simulink model "LKAS"  (R2018b)
settings: Solver=FixedStepDiscrete  StartTime=0.0  StopTime=10.0  FixedStep=0.01  RelTol=1e-3
InitFcn:
  | tmpVer = ver('MATLAB');
  | tmpVer = str2num(tmpVer.Version);
  | % -------------------------------------------------------------------
  | %  MATLAB file generated by Simulink.saveVars on 21-Nov-2019 10:06:14
  | %  MATLAB version: 7.13.0.564 (R2011b)
  | % -------------------------------------------------------------------
  | 
  | 
  | SInt16 = Simulink.AliasType;
  | SInt16.Description = 'Num';
  | if (tmpVer > 7.11)
  | 	SInt16.DataScope = 'Auto';
  | end
  | SInt16.HeaderFile = 'Rte_Type.h';
  | SInt16.BaseType = 'int16';
  | 
  | SInt32 = Simulink.AliasType;
  | SInt32.Description = 'Num';
  | if (tmpVer > 7.11)
  | 	SInt32.DataScope = 'Auto';
  | end
  | SInt32.HeaderFile = 'Rte_Type.h';
  | SInt32.BaseType = 'int32';
  | 
  | SInt8 = Simulink.AliasType;
  | SInt8.Description = 'Num';
  | if (tmpVer > 7.11)
  | 	SInt8.DataScope = 'Auto';
  | end
  | SInt8.HeaderFile = 'Rte_Type.h';
  | SInt8.BaseType = 'int8';
  | 
  | T_A_m2_1024_1_u32 = Simulink.NumericType;
  | T_A_m2_1024_1_u32.Description = 'm2 (square meters  (m2))';
  | if (tmpVer > 7.11)
  | 	T_A_m2_1024_1_u32.DataScope = 'Auto';
  | end
  | T_A_m2_1024_1_u32.HeaderFile = 'Rte_Type.h';
  | T_A_m2_1024_1_u32.DataTypeMode = 'Fixed-point: slope and bias scaling';
  | T_A_m2_1024_1_u32.SignednessBool = false;
  | T_A_m2_1024_1_u32.WordLength = 32;
  | T_A_m2_1024_1_u32.FixedExponent = -10;
  | T_A_m2_1024_1_u32.SlopeAdjustmentFactor = 1;
  | T_A_m2_1024_1_u32.Bias = 0;
  | T_A_m2_1024_1_u32.DataTypeOverride = 'Inherit';
  | T_A_m2_1024_1_u32.IsAlias = true;
  | 
  | T_A_m2_65536_1_u16 = Simulink.NumericType;
  | T_A_m2_65536_1_u16.Description = 'm2 (square meters  (m2))';
  | if (tmpVer > 7.11)
  | 	T_A_m2_65536_1_u16.DataScope = 'Auto';
  | end
  | T_A_m2_65536_1_u16.HeaderFile = 'Rte_Type.h';
  | T_A_m2_65536_1_u16.DataTypeMode = 'Fixed-point: slope and bias scaling';
  | T_A_m2_65536_1_u16.SignednessBool = false;
  | T_A_m2_65536_1_u16.WordLength = 16;
  | T_A_m2_65536_1_u16.FixedExponent = -16;
  | T_A_m2_65536_1_u16.SlopeAdjustmentFactor = 1;
  | T_A_m2_65536_1_u16.Bias = 0;
  | T_A_m2_65536_1_u16.DataTypeOverride = 'Inherit';
  | ... (+4598 lines)
StopFcn:
  | clear  T_A_m2_1024_1_u32 T_A_m2_65536_1_u16 T_A_m2_Float32 T_A_mm2_10_1_u16 T_A_mm2_4_1_s16 T_A_mm2_Float32 T_Cnt_Num_10_1_u32 T_Cnt_Num_1_1_s16 T_Cnt_Num_1_1_s32 T_Cnt_Num_1_1_s8 T_Cnt_Num_1_1_u16 T_Cnt_Num_1_1_u32 T_Cnt_Num_1_1_u8 T_E_J_1_1_s32 T_E_J_Float32 T_E_kJ_128_1_s32 T_E_kJ_Float32 T_E_kwh_10_1_u16 T_E_kwh_Float32 T_Epl_kwhpkm_100_1_u16 T_Epl_kwhpkm_Float32 T_F_N_1_1_s16 T_F_N_Float32 T_I_A_1000_1_u16 T_I_A_1048576_1_s32 T_I_A_2048_1_s16 T_I_A_32_1_s16 T_I_A_Float32 T_I_mA_1_1_s16 T_I_mA_32768_128_s16 T_I_mA_Float32 T_J_kgpm2_128_1_u16 T_J_kgpm2_Float32 T_K_NA_1000_1_s16 T_K_NA_100_1_s16 T_K_NA_100_1_u16 T_K_NA_1024_1_s16 T_K_NA_1024_1_u16 T_K_NA_128_1_s16 T_K_NA_128_1_u16 T_K_NA_128_1_u8 T_K_NA_16777216_1_u32 T_K_NA_16_1_s16 T_K_NA_16_1_u16 T_K_NA_16_1_u8 T_K_NA_1_16_u16 T_K_NA_1_1_s16 T_K_NA_1_1_u16 T_K_NA_1_1_u8 T_K_NA_32768_1_s16 T_K_NA_32768_1_u16 T_K_NA_32_1_s8 T_K_NA_4096_1_u16 T_K_NA_4194304_1_s32 T_K_NA_4194304_1_u16 T_K_NA_65536_1_s32 T_K_NA_65536_1_u16 T_K_NA_8192_1_s16 T_K_NA_8_1_s16 T_K_NA_Float32 T_M_Nm_16_1_s16 T_M_Nm_1_1_s16 T_M_Nm_32768_1_s16 T_M_Nm_32_1_s16 T_M_Nm_4_1_s16 T_M_Nm_512_1_s16 T_M_Nm_Float32 T_P_W_1_4_s16 T_P_W_1_8_s16 T_P_W_Float32 T_P_kW_128_1_s16 T_P_kW_1_8_s16 T_P_kW_8_1_s32 T_P_kW_Float32 T_Pct_pct_1024_1_s32 T_Pct_pct_1024_1_u32 T_Pct_pct_10_1_s16 T_Pct_pct_10_1_u32 T_Pct_pct_128_100_s8 T_Pct_pct_1_1_s16 T_Pct_pct_1_4_u8 T_Pct_pct_255_100_u16 T_Pct_pct_255_100_u8 T_Pct_pct_256_1_s16 T_Pct_pct_256_1_u16 T_Pct_pct_65535_100_u16 T_Pct_pct_Float32 T_R_ohm_1024_1_s16 T_R_ohm_32_1_s16 T_R_ohm_Float32 T_TK_K_16_1_s16 T_TK_K_Float32 T_T_degC_10_400_1_u16 T_T_degC_16_1_s16 T_T_degC_1_40_1_u8 T_T_degC_2_80_1_u8 T_T_degC_Float32 T_U_V_1000_1_u16 T_U_V_10_1_u8 T_U_V_200_1_u8 T_U_V_32_1_s16 T_U_V_4096_1_s16 T_U_V_512_1_s16 T_U_V_65535_8_u16 T_U_V_8192_1_u16 T_U_V_Float32 T_U_mV_1_1_s16 T_U_mV_256_20_u16 T_U_mV_Float32 T_V_l_256_1_s16 T_V_l_4096_1_s16 T_V_l_64_1_s16 T_V_l_65535_100_u16 T_V_l_Float32 T_V_ml_128_1_s16 T_V_ml_1_1_s16 T_V_ml_32768_1_s16 T_V_ml_Float32 T_V_ul_32_1_u16 T_V_ul_Float32 T_Vpl_clpkm_512_1_u16 T_Vpl_clpkm_Float32 T_a_kphps_16_1_s16 T_a_kphps_Float32 T_a_mps2_128_1_s16 T_a_mps2_Float32 T_c_MJpkg_256_1_s16 T_c_MJpkg_Float32 T_c_kJpgpK_1024_1_s16 T_c_kJpgpK_Float32 T_c_kJpkgpK_128_1_u16 T_c_kJpkgpK_Float32 T_chrg_Ah_1_1_s16 T_chrg_Ah_1_1_u16 T_chrg_Ah_1_1_u8 T_chrg_Ah_256_1_u16 T_chrg_Ah_4194304_1_s32 T_chrg_Ah_512_1_u16 T_chrg_Ah_8_1_u16 T_chrg_Ah_Float32 T_cmp_NA_100_1_s16 T_cmp_NA_128_1_s16 T_cmp_NA_16_1_s16 T_cmp_NA_32768_1_u16 T_cmp_NA_Float32 T_d2n_rpmps2_4_1_s16 T_d2n_rpmps2_Float32 T_dPct_pctps_16_1_s16 T_dPct_pctps_256_1_s16 T_dPct_pctps_Float32 T_dT_degCps_128_1_s16 T_dT_degCps_Float32 T_dV_lph_1_1_s16 T_dV_lph_Float32 T_dV_lpm_128_1_s16 T_dV_lpm_32_1_s16 T_dV_lpm_Float32 T_dV_lps_1024_1_u16 T_dV_lps_4_1_u16 T_dV_lps_Float32 T_dV_mlps_1024_1_s16 T_dV_mlps_Float32 T_d_BitField16 T_dm_gps_128_1_s16 T_dm_gps_128_1_u16 T_dm_gps_256_1_u16 T_dm_gps_Float32 T_dm_mgps_1_1_s16 T_dm_mgps_Float32 T_dn_rpmps_1_1_s16 T_dn_rpmps_2_1_s16 T_dn_rpmps_Float32 T_dp_Paps_1_1_s16 T_dp_Paps_Float32 T_dp_kPaps_1_1_s16 T_dp_kPaps_8_1_s16 T_dp_kPaps_Float32 T_dphi_degps_128_1_s16 T_dphi_degps_8_1_s16 T_dphi_degps_Float32 T_dr_ps_256_1_s16 T_dr_ps_Float32 T_drho_mgplps_1_2_s16 T_drho_mgplps_Float32 T_e_NA_1_1_u8 T_f_Hz_1_1_u16 T_f_Hz_1_1_u32 T_f_Hz_64_1_u16 T_f_Hz_8_1_s16 T_f_Hz_Float32 T_g_BitField32 T_l_km_16_1_s16 T_l_km_1_1_u16 T_l_km_1_1_u32 T_l_km_Float32 T_l_m_1024_1_s16 T_l_m_16_1_s16 T_l_m_1_1_u32 T_l_m_Float32 T_l_mm_16_1_s16 T_l_mm_1_1_u16 T_l_mm_4096_1_s16 T_l_mm_4_1_u8 T_l_mm_64_1_s16 T_l_mm_Float32 T_m_g_1_1_s16 T_m_g_2048_1_s16 T_m_g_32_1_u16 T_m_g_Float32 T_m_kg_1024_1_s16 T_m_kg_1_1_s16 T_m_kg_1_1_u32 T_m_kg_Float32 T_m_mg_128_1_s16 T_m_mg_32_1_s16 T_m_mg_Float32 T_n_rpm_1_1_s16 T_n_rpm_1_25_u8 T_n_rpm_256_50_u16 T_n_rpm_2_25_u8 T_n_rpm_4_1_u16 T_n_rpm_Float32 T_p_MPa_64_1_s16 T_p_MPa_Float32 T_p_Pa_1_1_s16 T_p_Pa_Float32 T_p_kPa_1_10_u16 T_p_kPa_1_1_s16 T_p_kPa_1_1_u8 T_p_kPa_256_1_u16 T_p_kPa_32_1_u16 T_p_kPa_64_1_s16 T_p_kPa_Float32 T_phi_deg_100_1_s16 T_phi_deg_1024_1_s16 T_phi_deg_128_1_s16 T_phi_deg_1_1_u8 T_phi_deg_256_1_s16 T_phi_deg_2_1_s8 T_phi_deg_32_1_s16 T_phi_deg_512_6_s32 T_phi_deg_Float32 T_phi_rad_2048_1_s16 T_phi_rad_Float32 T_r_NA_1024_1_s16 T_r_NA_1024_1_u16 T_r_NA_16384_1_s16 T_r_NA_16_1_s16 T_r_NA_256_1_s8 T_r_NA_256_1_u16 T_r_NA_32768_1_u16 T_r_NA_32_1_u16 T_r_NA_4096_1_s16 T_r_NA_65535_2_u16 T_r_NA_8192_1_u16 T_r_NA_Float32 T_rho_gpl_8192_1_s16 T_rho_gpl_Float32 T_rho_kgpm3_16_1_s16 T_rho_kgpm3_Float32 T_rho_mgpl_1_1_s16 T_rho_mgpl_64_1_s16 T_rho_mgpl_Float32 T_t_hour_1_1_s16 T_t_hour_Float32 T_t_m_1_1_u16 T_t_m_Float32 T_t_ms_1_1_s16 T_t_ms_1_1_u16 T_t_ms_1_1_u32 T_t_ms_4096_1_s16 T_t_ms_64_1_s16 T_t_ms_Float32 T_t_s_1000_1_s16 T_t_s_100_1_s16 T_t_s_10_1_s16 T_t_s_10_1_u16 T_t_s_1_1_s16 T_t_s_1_1_u16 T_t_s_1_1_u32 T_t_s_Float32 T_t_us_10_1_u32 T_t_us_1_1_s16 T_t_us_1_1_u32 T_t_us_1_4_u16 T_t_us_Float32 T_v_kph_1_1_u8 T_v_kph_64_1_s16 T_v_kph_64_1_u16 T_v_kph_Float32 T_v_mps_256_1_s16 T_v_mps_Float32 T_w_radps_32_1_s16 T_w_radps_Float32 T_y_BitField8 T_y_BitFieldDiagProgress T_y_BitFieldDiagStatus T_y_NA_1_1_u8 SInt16 SInt32 SInt8 T_BOOLEAN UInt16 UInt32 UInt8 s16 s32 s8 u16 u32 u8
model workspace (MAT data in the model file):
  MCOS : class17 (value not decoded)
  MCOS : class17 (value not decoded)
  MCOS : class17 (value not decoded)
  MCOS : class17 (value not decoded)
  MCOS : class17 (value not decoded)
  MCOS : class17 (value not decoded)
  MCOS : class17 (value not decoded)
  MCOS : class17 (value not decoded)
  MCOS : class17 (value not decoded)
  MCOS : class17 (value not decoded)
  MCOS : class17 (value not decoded)
  MCOS : class17 (value not decoded)
  MCOS : class17 (value not decoded)
  MCOS : class17 (value not decoded)
  MCOS : class17 (value not decoded)
  MCOS : class17 (value not decoded)
  MCOS : class17 (value not decoded)
  MCOS : class17 (value not decoded)
  MCOS : class17 (value not decoded)
  MCOS : class17 (value not decoded)
  MCOS : class17 (value not decoded)
  MCOS : class17 (value not decoded)
  MCOS : class17 (value not decoded)
  MCOS : class17 (value not decoded)
  MCOS : class17 (value not decoded)
  MCOS : class17 (value not decoded)
  MCOS : class17 (value not decoded)
  MCOS : class17 (value not decoded)
  MCOS : class17 (value not decoded)
  MCOS : class17 (value not decoded)
  MCOS : class17 (value not decoded)
  MCOS : class17 (value not decoded)
  MCOS : class17 (value not decoded)
  MCOS : class17 (value not decoded)
  MCOS : class17 (value not decoded)
  MCOS : class17 (value not decoded)
  MCOS : class17 (value not decoded)
  MCOS : class17 (value not decoded)
  MCOS : class17 (value not decoded)
  MCOS : class17 (value not decoded)
  MCOS : class17 (value not decoded)
  MCOS : class17 (value not decoded)
  MCOS : class17 (value not decoded)
  MCOS : class17 (value not decoded)
  MCOS : class17 (value not decoded)
  MCOS : class17 (value not decoded)
  MCOS : class17 (value not decoded)
  MCOS : class17 (value not decoded)
  MCOS : class17 (value not decoded)
  MCOS : class17 (value not decoded)
  MCOS : class17 (value not decoded)
  MCOS : class17 (value not decoded)
  MCOS : class17 (value not decoded)
  MCOS : class17 (value not decoded)
  MCOS : class17 (value not decoded)
  MCOS : class17 (value not decoded)
  MCOS : class17 (value not decoded)
  MCOS : class17 (value not decoded)
  MCOS : class17 (value not decoded)
  MCOS : class17 (value not decoded)
  MCOS : class17 (value not decoded)
  MCOS : class17 (value not decoded)
  MCOS : class17 (value not decoded)
  MCOS : class17 (value not decoded)
  MCOS : class17 (value not decoded)
  MCOS : class17 (value not decoded)
  MCOS : class17 (value not decoded)
  MCOS : class17 (value not decoded)
  MCOS : class17 (value not decoded)
  MCOS : class17 (value not decoded)
  MCOS : class17 (value not decoded)
  MCOS : class17 (value not decoded)
  MCOS : class17 (value not decoded)
  MCOS : class17 (value not decoded)
  MCOS : class17 (value not decoded)
  MCOS : class17 (value not decoded)
  MCOS : class17 (value not decoded)
  MCOS : class17 (value not decoded)
  MCOS : class17 (value not decoded)
  MCOS : class17 (value not decoded)
  MCOS : class17 (value not decoded)
  MCOS : class17 (value not decoded)
  MCOS : class17 (value not decoded)
  MCOS : class17 (value not decoded)
  MCOS : class17 (value not decoded)
  MCOS : class17 (value not decoded)
  MCOS : class17 (value not decoded)
  MCOS : class17 (value not decoded)
  MCOS : class17 (value not decoded)
undefined symbols (not defined in the file): LKA_CarWidth, LKA_SampleTime, LKA_StrRatio_C, LKA_Veh2CamL_C, LKA_Veh2CamW_C, LKA_WhlBaseL_C, LL_CompSWA_C, LL_CrvtPrvwT_C, LL_DesDvt_C, LL_DvtComp_C, LL_DvtPrvwT_C, LL_DvtSpdDet_vDvtSpdMin_C, LL_HdAgExT_C, LL_HdAgPrvwT_C, LL_LAccMax_C, LL_LAccRMax_C, LL_LDW_EarliestWarnLine_C, LL_LDW_LatestWarnLine_C, LL_LDWS_SUPPRESS_HEADING, LL_LFClb_TFC_DiffCtlBalance, LL_LFClb_TFC_DiffCtrlMaxSWA, LL_LFClb_TFC_DiffCtrlRatio, LL_LFClb_TFC_facmGainLutGain1_C, LL_LFClb_TFC_facmGainLutGain2_C, LL_LFClb_TFC_facmIntegRatio, LL_LFClb_TFC_facmKlat_C, LL_LFClb_TFC_FfCtlRatio_C, LL_LFClb_TFC_phiIntegCtlMaxSWA_C, LL_LFClb_TFC_tiKlatPrvwT_C, LL_LFClb_TFC_vGainLutVehSpdLwr_C, LL_LFClb_TFC_vGainLutVehSpdUpr_C, LL_LKA_EarliestWarnLine_C, LL_LKA_LatestWarnLine_C, LL_LKAExPrcs_ExitC0Dvt, LL_LKAExPrcs_ExitC0Swt, LL_LKAExPrcs_tiExitTime1, LL_LKAExPrcs_tiExitTime2, LL_LKAExPrcs_tiExitTime3, LL_LKAS_OUT_OF_CONTROL_LAT_VEL, LL_LKAS_OUT_OF_CONTROL_TTLC, LL_LKASWASyn_M0, LL_LKASWASyn_M1, LL_LKASWASyn_M2, LL_LKASWASyn_M3K, LL_LKASWASyn_SWAaddMax, LL_LKASWASyn_T2, LL_LKASWASyn_tiTrqSwaRtTime, LL_LKASWASyn_tiTrqSwaTime, LL_LKASWASyn_TrqMax, LL_LKASWASyn_TrqSwaAddSwt, LL_LKASWASyn_TrqSwaRateDiff, LL_LSpdCompT_C, LL_lStpLngth_C, LL_MAX_DELAY_EPSSTAR_TIME, LL_MAX_DRIVER_TORQUE_DISABLE, LL_MAX_DRIVER_TORQUE_ENABLE, LL_MAX_LANE_WIDTH_DISABLE, LL_MAX_LANE_WIDTH_ENABLE, LL_MAX_LAT_ACC_DISABLE, LL_MAX_LAT_ACC_ENABLE ... (+29)
libraries: simulink x134, dspstat3 x3, simulink_extras x1
(part 4 of 18)

== system LKAS/LKAS/Output ==
  bsLLOut : Inport
  Bus Selector : BusSelector  OutputSignals=Vehicle_Lane_Display,LDW_Status_Display,LKA_Status_Display,LDW_Flag,Hands_off_warning,LKA_action_indication,HMI_Popup_Status,EPS_State_Ctl,LMS_phiSWACmd,Coefficient_toregulate_EPS,Permit_to_know_if_LKA_or_LPA3F2
  Cast To Single{1..9} (9 alike) : DataTypeConversion  OutDataTypeStr=UInt8
  Cast To Single10 : DataTypeConversion  OutDataTypeStr=T_M_Nm_Float32
  Cast To Single11 : DataTypeConversion  OutDataTypeStr=T_M_Nm_Float32
  Vehicle_Lane_Display : Outport
  LDW_Status_Display : Outport  Port=2
  LKA_Status_Display : Outport  Port=3
  LDW_Flag : Outport  Port=4
  Hands_Off_Warning : Outport  Port=5
  LKA_Action_Indication : Outport  Port=6
  HMI_Popup_Status : Outport  Port=7
  EPS_State_Control : Outport  Port=8
  LKA_SWA_Control : Outport  Port=9
  EPS_Factor_Control : Outport  Port=10
  EPS_LKA_Control : Outport  Port=11
  wires:
  bsLLOut/1 -> Bus Selector/1  "bsLLOutput"
  Bus Selector/1 -> Cast To Single1/1  "<Vehicle_Lane_Display>"
  Bus Selector/2 -> Cast To Single2/1  "<LDW_Status_Display>"
  Bus Selector/3 -> Cast To Single3/1  "<LKA_Status_Display>"
  Bus Selector/4 -> Cast To Single4/1  "<LDW_Flag>"
  Bus Selector/5 -> Cast To Single5/1  "<Hands_off_warning>"
  Bus Selector/6 -> Cast To Single6/1  "<LKA_action_indication>"
  Bus Selector/7 -> Cast To Single7/1  "<HMI_Popup_Status>"
  Bus Selector/8 -> Cast To Single8/1  "<EPS_State_Ctl>"
  Bus Selector/9 -> Cast To Single11/1  "<LMS_phiSWACmd>"
  Bus Selector/10 -> Cast To Single10/1  "<Coefficient_toregulate_EPS>"
  Bus Selector/11 -> Cast To Single9/1  "<Permit_to_know_if_LKA_or_LPA3F2>"
  Cast To Single1/1 -> Vehicle_Lane_Display/1  "Vehicle_Lane_Display"
  Cast To Single2/1 -> LDW_Status_Display/1  "LDW_Status_Display"
  Cast To Single3/1 -> LKA_Status_Display/1  "LKA_Status_Display"
  Cast To Single4/1 -> LDW_Flag/1  "LDW_Flag"
  Cast To Single5/1 -> Hands_Off_Warning/1  "Hands_Off_Warning"
  Cast To Single6/1 -> LKA_Action_Indication/1  "LKA_Action_Indication"
  Cast To Single7/1 -> HMI_Popup_Status/1  "HMI_Popup_Status"
  Cast To Single8/1 -> EPS_State_Control/1  "EPS_State_Control"
  Cast To Single9/1 -> EPS_LKA_Control/1  "EPS_LKA_Control"
  Cast To Single10/1 -> EPS_Factor_Control/1  "EPS_Factor_Control"
  Cast To Single11/1 -> LKA_SWA_Control/1  "LKA_SWA_Control"

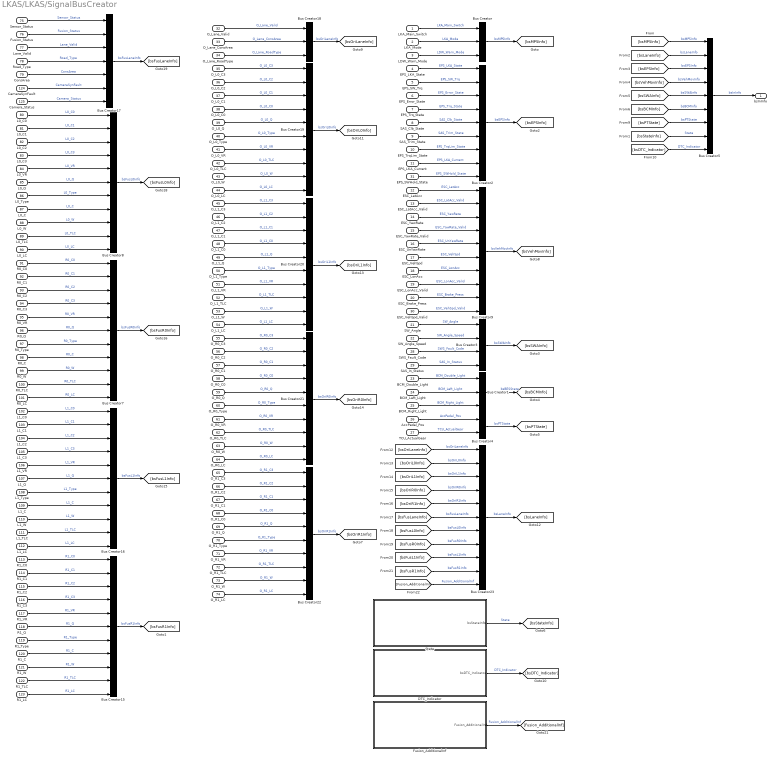
== system LKAS/LKAS/SignalBusCreator ==
  LKA_Main_Switch : Inport
  LKA_Mode : Inport  Port=2
  LDW_Warn_Mode : Inport  Port=3
  EPS_LKA_State : Inport  Port=4
  EPS_SW_Trq : Inport  Port=5
  EPS_Error_State : Inport  Port=6
  EPS_Trq_State : Inport  Port=7
  SAS_Clb_State : Inport  Port=8
  SAS_Trim_State : Inport  Port=9
  EPS_TrqLim_State : Inport  Port=10
  EPS_LKA_Current : Inport  Port=11
  ESC_LatAcc : Inport  Port=12
  ESC_LatAcc_Valid : Inport  Port=13
  ESC_YawRate : Inport  Port=14
  ESC_YawRate_Valid : Inport  Port=15
  ESC_UnYawRate : Inport  Port=16
  ESC_VehSpd : Inport  Port=17
  ESC_LonAcc : Inport  Port=18
  ESC_LonAcc_Valid : Inport  Port=19
  ESC_Brake_Press : Inport  Port=20
  SW_Angle : Inport  Port=21
  SW_Angle_Speed : Inport  Port=22
  BCM_Double_Light : Inport  Port=23
  BCM_Left_Light : Inport  Port=24
  BCM_Right_Light : Inport  Port=25
  AccPedal_Pos : Inport  Port=26
  TCU_ActualGear : Inport  Port=27
  SWS_Fault_Code : Inport  Port=28
  SAS_In_Status : Inport  Port=29
  ESC_VehSpd_Valid : Inport  Port=30
  EPS_SWHold_State : Inport  Port=31
  O_Lane_Valid : Inport  Port=32
  O_Lane_ConsArea : Inport  Port=33
  O_Lane_RoadType : Inport  Port=34
  O_L0_C3 : Inport  Port=35
  O_L0_C2 : Inport  Port=36
  O_L0_C1 : Inport  Port=37
  O_L0_C0 : Inport  Port=38
  O_L0_Q : Inport  Port=39
  O_L0_Type : Inport  Port=40
  O_L0_VR : Inport  Port=41
  O_L0_TLC : Inport  Port=42
  O_L0_W : Inport  Port=43
  O_L0_LC : Inport  Port=44
  O_L1_C3 : Inport  Port=45
  O_L1_C2 : Inport  Port=46
  O_L1_C1 : Inport  Port=47
  O_L1_C0 : Inport  Port=48
  O_L1_Q : Inport  Port=49
  O_L1_Type : Inport  Port=50
  O_L1_VR : Inport  Port=51
  O_L1_TLC : Inport  Port=52
  O_L1_W : Inport  Port=53
  O_L1_LC : Inport  Port=54
  O_R0_C3 : Inport  Port=55
  O_R0_C2 : Inport  Port=56
  O_R0_C1 : Inport  Port=57
  O_R0_C0 : Inport  Port=58
  O_R0_Q : Inport  Port=59
  O_R0_Type : Inport  Port=60
  O_R0_VR : Inport  Port=61
  O_R0_TLC : Inport  Port=62
  O_R0_W : Inport  Port=63
  O_R0_LC : Inport  Port=64
  O_R1_C3 : Inport  Port=65
  O_R1_C2 : Inport  Port=66
  O_R1_C1 : Inport  Port=67
  O_R1_C0 : Inport  Port=68
  O_R1_Q : Inport  Port=69
  O_R1_Type : Inport  Port=70
  O_R1_VR : Inport  Port=71
  O_R1_TLC : Inport  Port=72
  O_R1_W : Inport  Port=73
  O_R1_LC : Inport  Port=74
  Sensor_Status : Inport  Port=75
  Fusion_Status : Inport  Port=76
  Lane_Valid : Inport  Port=77
  Road_Type : Inport  Port=78
  ConsArea : Inport  Port=79
  L0_C0 : Inport  Port=80
  L0_C1 : Inport  Port=81
  L0_C2 : Inport  Port=82
  L0_C3 : Inport  Port=83
  L0_VR : Inport  Port=84
  L0_Q : Inport  Port=85
  L0_Type : Inport  Port=86
  L0_C : Inport  Port=87
  L0_W : Inport  Port=88
  L0_TLC : Inport  Port=89
  L0_LC : Inport  Port=90
  R0_C0 : Inport  Port=91
  R0_C1 : Inport  Port=92
  R0_C2 : Inport  Port=93
  R0_C3 : Inport  Port=94
  R0_VR : Inport  Port=95
  R0_Q : Inport  Port=96
  R0_Type : Inport  Port=97
  R0_C : Inport  Port=98
  R0_W : Inport  Port=99
  R0_TLC : Inport  Port=100
  R0_LC : Inport  Port=101
  L1_C0 : Inport  Port=102
  L1_C1 : Inport  Port=103
  L1_C2 : Inport  Port=104
  L1_C3 : Inport  Port=105
  L1_VR : Inport  Port=106
  L1_Q : Inport  Port=107
  L1_Type : Inport  Port=108
  L1_C : Inport  Port=109
  L1_W : Inport  Port=110
  L1_TLC : Inport  Port=111
  L1_LC : Inport  Port=112
  R1_C0 : Inport  Port=113
  R1_C1 : Inport  Port=114
  R1_C2 : Inport  Port=115
  R1_C3 : Inport  Port=116
  R1_VR : Inport  Port=117
  R1_Q : Inport  Port=118
  R1_Type : Inport  Port=119
  R1_C : Inport  Port=120
  R1_W : Inport  Port=121
  R1_TLC : Inport  Port=122
  R1_LC : Inport  Port=123
  CameraSynFault : Inport  Port=124
  Camera_Status : Inport  Port=125
  Bus Creator : BusCreator  Inputs=3
  Bus Creator1 : BusCreator  Inputs=3
  Bus Creator{7..8,15..16,23} (5 alike) : BusCreator  Inputs=11
  Bus Creator17 : BusCreator  Inputs=7
  Bus Creator18 : BusCreator  Inputs=3
  Bus Creator{9,19..22} (5 alike) : BusCreator  Inputs=10
  Bus Creator2 : BusCreator  Inputs=9
  Bus Creator3 : BusCreator  Inputs=4
  Bus Creator4 : BusCreator  Inputs=2
  Bus Creator5 : BusCreator  Inputs=9
  DTC_Indicator : Subsystem
  Fusion_AdditionalInf : Subsystem
  State : Subsystem
  bsInInfo : Outport
  wires:
  Bus Creator9/1 -> [bsVehMovInfo]  "bsVehMovInfo"
  Bus Creator3/1 -> [bsSWAInfo]  "bsSWAInfo"
  Bus Creator1/1 -> [bsBCMInfo]  "bsBESState"
  Bus Creator2/1 -> [bsEPSInfo]  "bsEPSInfo"
  Bus Creator/1 -> [bsMP5Info]  "bsMP5Info"
  [bsLaneInfo] -> Bus Creator5/2  "bsLaneInfo"
  [bsEPSInfo] -> Bus Creator5/3  "bsEPSInfo"
  [bsVehMovInfo] -> Bus Creator5/4  "bsVehMovInfo"
  [bsSWAInfo] -> Bus Creator5/5  "bsSWAInfo"
  [bsBCMInfo] -> Bus Creator5/6  "bsBCMInfo"
  [bsPTState] -> Bus Creator5/7  "bsPTState"
  [bsMP5Info] -> Bus Creator5/1  "bsMP5Info"
  [bsStateInfo] -> Bus Creator5/8  "State"
  [bsDTC_Indicator] -> Bus Creator5/9  "DTC_Indicator"
  Bus Creator4/1 -> [bsPTState]  "bsPTState"
  Bus Creator7/1 -> [bsFusR0Info]  "bsFusR0Info"
  Bus Creator16/1 -> [bsFusL1Info]  "bsFusL1Info"
  Bus Creator15/1 -> [bsFusR1Info]  "bsFusR1Info"
  Bus Creator17/1 -> [bsFusLaneInfo]  "bsFusLaneInfo"
  Bus Creator18/1 -> [bsOriLaneInfo]  "bsOriLaneInfo"
  Bus Creator19/1 -> [bsOriL0Info]  "bsOriL0Info"
  Bus Creator20/1 -> [bsOriL1Info]  "bsOriL1Info"
  Bus Creator22/1 -> [bsOriR1Info]  "bsOriR1Info"
  Bus Creator21/1 -> [bsOriR0Info]  "bsOriR0Info"
  Bus Creator8/1 -> [bsFusL0Info]  "bsFusL0Info"
  [bsOriLaneInfo] -> Bus Creator23/1  "bsOriLaneInfo"
  [bsOriL0Info] -> Bus Creator23/2  "bsOriL0Info"
  [bsOriL1Info] -> Bus Creator23/3  "bsOriL1Info"
  [bsOriR0Info] -> Bus Creator23/4  "bsOriR0Info"
  [bsOriR1Info] -> Bus Creator23/5  "bsOriR1Info"
  [bsFusLaneInfo] -> Bus Creator23/6  "bsFusLaneInfo"
  [bsFusL0Info] -> Bus Creator23/7  "bsFusL0Info"
  [bsFusR0Info] -> Bus Creator23/8  "bsFusR0Info"
  [bsFusL1Info] -> Bus Creator23/9  "bsFusL1Info"
  [bsFusR1Info] -> Bus Creator23/10  "bsFusR1Info"
  Bus Creator23/1 -> [bsLaneInfo]  "bsLaneInfo"
  [Fusion_AdditionalInf] -> Bus Creator23/11  "Fusion_AdditionalInf"
  DTC_Indicator/1(bsDTC_Indicator) -> [bsDTC_Indicator]  "DTC_Indicator"
  State/1(bsStateInfo) -> [bsStateInfo]  "State"
  Bus Creator5/1 -> bsInInfo/1  "bsInInfo"
  Fusion_AdditionalInf/1(Fusion_AdditionalInf) -> [Fusion_AdditionalInf]  "Fusion_AdditionalInf"
  AccPedal_Pos/1 -> Bus Creator4/1  "AccPedal_Pos"
  TCU_ActualGear/1 -> Bus Creator4/2  "TCU_ActualGear"
  BCM_Double_Light/1 -> Bus Creator1/1  "BCM_Double_Light"
  BCM_Left_Light/1 -> Bus Creator1/2  "BCM_Left_Light"
  BCM_Right_Light/1 -> Bus Creator1/3  "BCM_Right_Light"
  SW_Angle/1 -> Bus Creator3/1  "SW_Angle"
  SW_Angle_Speed/1 -> Bus Creator3/2  "SW_Angle_Speed"
  SWS_Fault_Code/1 -> Bus Creator3/3  "SWS_Fault_Code"
  SAS_In_Status/1 -> Bus Creator3/4  "SAS_In_Status"
  ESC_LatAcc/1 -> Bus Creator9/1  "ESC_LatAcc"
  ESC_LatAcc_Valid/1 -> Bus Creator9/2  "ESC_LatAcc_Valid"
  ESC_YawRate/1 -> Bus Creator9/3  "ESC_YawRate"
  ESC_YawRate_Valid/1 -> Bus Creator9/4  "ESC_YawRate_Valid"
  ESC_UnYawRate/1 -> Bus Creator9/5  "ESC_UnYawRate"
  ESC_VehSpd/1 -> Bus Creator9/6  "ESC_VehSpd"
  ESC_LonAcc/1 -> Bus Creator9/7  "ESC_LonAcc"
  ESC_LonAcc_Valid/1 -> Bus Creator9/8  "ESC_LonAcc_Valid"
  ESC_Brake_Press/1 -> Bus Creator9/9  "ESC_Brake_Press"
  ESC_VehSpd_Valid/1 -> Bus Creator9/10  "ESC_VehSpd_Valid"
  EPS_LKA_State/1 -> Bus Creator2/1  "EPS_LKA_State"
  EPS_SW_Trq/1 -> Bus Creator2/2  "EPS_SW_Trq"
  EPS_Error_State/1 -> Bus Creator2/3  "EPS_Error_State"
  EPS_Trq_State/1 -> Bus Creator2/4  "EPS_Trq_State"
  SAS_Clb_State/1 -> Bus Creator2/5  "SAS_Clb_State"
  SAS_Trim_State/1 -> Bus Creator2/6  "SAS_Trim_State"
  EPS_TrqLim_State/1 -> Bus Creator2/7  "EPS_TrqLim_State"
  EPS_LKA_Current/1 -> Bus Creator2/8  "EPS_LKA_Current"
  EPS_SWHold_State/1 -> Bus Creator2/9  "EPS_SWHold_State"
  LKA_Main_Switch/1 -> Bus Creator/1  "LKA_Main_Switch"
  LKA_Mode/1 -> Bus Creator/2  "LKA_Mode"
  LDW_Warn_Mode/1 -> Bus Creator/3  "LDW_Warn_Mode"
  O_Lane_Valid/1 -> Bus Creator18/1  "O_Lane_Valid"
  O_Lane_ConsArea/1 -> Bus Creator18/2  "O_Lane_ConsArea"
  O_Lane_RoadType/1 -> Bus Creator18/3  "O_Lane_RoadType"
  O_L0_C3/1 -> Bus Creator19/1  "O_L0_C3"
  O_L0_C2/1 -> Bus Creator19/2  "O_L0_C2"
  O_L0_C1/1 -> Bus Creator19/3  "O_L0_C1"
  O_L0_C0/1 -> Bus Creator19/4  "O_L0_C0"
  O_L0_Q/1 -> Bus Creator19/5  "O_L0_Q"
  O_L0_Type/1 -> Bus Creator19/6  "O_L0_Type"
  O_L0_VR/1 -> Bus Creator19/7  "O_L0_VR"
  O_L0_TLC/1 -> Bus Creator19/8  "O_L0_TLC"
  O_L0_W/1 -> Bus Creator19/9  "O_L0_W"
  O_L0_LC/1 -> Bus Creator19/10  "O_L0_LC"
  O_L1_C3/1 -> Bus Creator20/1  "O_L1_C3"
  O_L1_C2/1 -> Bus Creator20/2  "O_L1_C2"
  O_L1_C1/1 -> Bus Creator20/3  "O_L1_C1"
  O_L1_C0/1 -> Bus Creator20/4  "O_L1_C0"
  O_L1_Q/1 -> Bus Creator20/5  "O_L1_Q"
  O_L1_Type/1 -> Bus Creator20/6  "O_L1_Type"
  O_L1_VR/1 -> Bus Creator20/7  "O_L1_VR"
  O_L1_TLC/1 -> Bus Creator20/8  "O_L1_TLC"
  O_L1_W/1 -> Bus Creator20/9  "O_L1_W"
  O_L1_LC/1 -> Bus Creator20/10  "O_L1_LC"
  O_R0_C3/1 -> Bus Creator21/1  "O_R0_C3"
  O_R0_C2/1 -> Bus Creator21/2  "O_R0_C2"
  O_R0_C1/1 -> Bus Creator21/3  "O_R0_C1"
  O_R0_C0/1 -> Bus Creator21/4  "O_R0_C0"
  O_R0_Q/1 -> Bus Creator21/5  "O_R0_Q"
  O_R0_Type/1 -> Bus Creator21/6  "O_R0_Type"
  O_R0_VR/1 -> Bus Creator21/7  "O_R0_VR"
  O_R0_TLC/1 -> Bus Creator21/8  "O_R0_TLC"
  O_R0_W/1 -> Bus Creator21/9  "O_R0_W"
  O_R0_LC/1 -> Bus Creator21/10  "O_R0_LC"
  O_R1_C3/1 -> Bus Creator22/1  "O_R1_C3"
  O_R1_C2/1 -> Bus Creator22/2  "O_R1_C2"
  O_R1_C1/1 -> Bus Creator22/3  "O_R1_C1"
  O_R1_C0/1 -> Bus Creator22/4  "O_R1_C0"
  O_R1_Q/1 -> Bus Creator22/5  "O_R1_Q"
  O_R1_Type/1 -> Bus Creator22/6  "O_R1_Type"
  O_R1_VR/1 -> Bus Creator22/7  "O_R1_VR"
  O_R1_TLC/1 -> Bus Creator22/8  "O_R1_TLC"
  O_R1_W/1 -> Bus Creator22/9  "O_R1_W"
  O_R1_LC/1 -> Bus Creator22/10  "O_R1_LC"
  Sensor_Status/1 -> Bus Creator17/1  "Sensor_Status"
  Fusion_Status/1 -> Bus Creator17/2  "Fusion_Status"
  Lane_Valid/1 -> Bus Creator17/3  "Lane_Valid"
  Road_Type/1 -> Bus Creator17/4  "Road_Type"
  ConsArea/1 -> Bus Creator17/5  "ConsArea"
  CameraSynFault/1 -> Bus Creator17/6  "CameraSynFault"
  Camera_Status/1 -> Bus Creator17/7  "Camera_Status"
  L0_C0/1 -> Bus Creator8/1  "L0_C0"
  L0_C1/1 -> Bus Creator8/2  "L0_C1"
  L0_C2/1 -> Bus Creator8/3  "L0_C2"
  L0_C3/1 -> Bus Creator8/4  "L0_C3"
  L0_VR/1 -> Bus Creator8/5  "L0_VR"
  L0_Q/1 -> Bus Creator8/6  "L0_Q"
  L0_Type/1 -> Bus Creator8/7  "L0_Type"
  L0_C/1 -> Bus Creator8/8  "L0_C"
  L0_W/1 -> Bus Creator8/9  "L0_W"
  L0_TLC/1 -> Bus Creator8/10  "L0_TLC"
  L0_LC/1 -> Bus Creator8/11  "L0_LC"
  R0_C0/1 -> Bus Creator7/1  "R0_C0"
  R0_C1/1 -> Bus Creator7/2  "R0_C1"
  R0_C2/1 -> Bus Creator7/3  "R0_C2"
  R0_C3/1 -> Bus Creator7/4  "R0_C3"
  R0_VR/1 -> Bus Creator7/5  "R0_VR"
  R0_Q/1 -> Bus Creator7/6  "R0_Q"
  R0_Type/1 -> Bus Creator7/7  "R0_Type"
  R0_C/1 -> Bus Creator7/8  "R0_C"
  R0_W/1 -> Bus Creator7/9  "R0_W"
  R0_TLC/1 -> Bus Creator7/10  "R0_TLC"
  R0_LC/1 -> Bus Creator7/11  "R0_LC"
  L1_C0/1 -> Bus Creator16/1  "L1_C0"
  L1_C1/1 -> Bus Creator16/2  "L1_C1"
  L1_C2/1 -> Bus Creator16/3  "L1_C2"
  L1_C3/1 -> Bus Creator16/4  "L1_C3"
  L1_VR/1 -> Bus Creator16/5  "L1_VR"
  L1_Q/1 -> Bus Creator16/6  "L1_Q"
  L1_Type/1 -> Bus Creator16/7  "L1_Type"
  L1_C/1 -> Bus Creator16/8  "L1_C"
  L1_W/1 -> Bus Creator16/9  "L1_W"
  L1_TLC/1 -> Bus Creator16/10  "L1_TLC"
  L1_LC/1 -> Bus Creator16/11  "L1_LC"
  R1_C0/1 -> Bus Creator15/1  "R1_C0"
  R1_C1/1 -> Bus Creator15/2  "R1_C1"
  R1_C2/1 -> Bus Creator15/3  "R1_C2"
  R1_C3/1 -> Bus Creator15/4  "R1_C3"
  R1_VR/1 -> Bus Creator15/5  "R1_VR"
  R1_Q/1 -> Bus Creator15/6  "R1_Q"
  R1_Type/1 -> Bus Creator15/7  "R1_Type"
  R1_C/1 -> Bus Creator15/8  "R1_C"
  R1_W/1 -> Bus Creator15/9  "R1_W"
  R1_TLC/1 -> Bus Creator15/10  "R1_TLC"
  R1_LC/1 -> Bus Creator15/11  "R1_LC"

== system LKAS/LKAS/LL/Fault_Diagnostic ==
  bsInInfo : Inport
  Bus Creator : BusCreator  Inputs=2
  Bus Creator1 : BusCreator  Inputs=12
  Bus Selector3 : BusSelector  OutputSignals=DTC_Indicator.LKAS_BSWDTC_Status
  Bus Selector4 : BusSelector  OutputSignals=bsVehMovInfo.ESC_VehSpd_Valid,bsEPSInfo.EPS_LKA_State,bsEPSInfo.EPS_Error_State,bsEPSInfo.SAS_Clb_State,bsEPSInfo.SAS_Trim_State,bsSWAInfo.SWS_Fault_Code,bsSWAInfo.SAS_In_Status,bsPTState.TCU_ActualGear,bsEPSInfo.EPS_TrqLim_State,bsEPSInfo.EPS_Trq_State,bsVehMovInfo.ESC_LatAcc_Valid,bsVehMovInfo.ESC_YawRate_Valid,bsVehMovInfo.ESC_LonAcc_Valid
  Compare To Constant26 : simulink/Logic and Bit Operations/Compare To Constant  relop=~=  const=1  OutDataTypeStr=boolean
  Compare To Constant27 : simulink/Logic and Bit Operations/Compare To Constant  relop===  const=4  OutDataTypeStr=boolean
  Compare To Constant{28,30,36..39} (6 alike) : simulink/Logic and Bit Operations/Compare To Constant  relop===  const=1  OutDataTypeStr=boolean
  Compare To Constant29 : simulink/Logic and Bit Operations/Compare To Constant  relop===  const=0  OutDataTypeStr=boolean
  Compare To Constant31 : simulink/Logic and Bit Operations/Compare To Constant  relop===  const=2  OutDataTypeStr=boolean
  Compare To Constant32 : simulink/Logic and Bit Operations/Compare To Constant  relop=~=  const=0  OutDataTypeStr=boolean
  Compare To Constant33 : simulink/Logic and Bit Operations/Compare To Constant  relop=~=  const=1  OutDataTypeStr=boolean
  Compare To Constant34 : simulink/Logic and Bit Operations/Compare To Constant  relop=>  const=3  OutDataTypeStr=boolean
  Compare To Constant35 : simulink/Logic and Bit Operations/Compare To Constant  relop===  const=0  OutDataTypeStr=boolean
  Logical Operator5 : Logic  Operator=OR  AllPortsSameDT=off  OutDataTypeStr=boolean
  Logical Operator6 : Logic  Operator=OR  AllPortsSameDT=off  OutDataTypeStr=boolean
  bsSignalFault : Outport
  wires:
  Bus Creator/1 -> bsSignalFault/1
  Bus Selector3/1 -> Bus Creator/1  "<LKAS_BSWDTC_Status>"
  bsInInfo/1 -> Bus Selector4/1, Bus Selector3/1
  Bus Selector4/1 -> Compare To Constant26/1  "<ESC_VehSpd_Valid>"
  Compare To Constant26/1 -> Bus Creator1/1  "Event_FaulVehSpeed"
  Bus Selector4/2 -> Compare To Constant27/1  "<EPS_LKA_State>"
  Bus Selector4/4 -> Compare To Constant29/1  "<SAS_Clb_State>"
  Compare To Constant29/1 -> Bus Creator1/4  "Event_FaulSASClb"
  Bus Selector4/5 -> Compare To Constant30/1  "<SAS_Trim_State>"
  Bus Selector4/6 -> Compare To Constant32/1  "<SWS_Fault_Code>"
  Bus Selector4/7 -> Compare To Constant33/1  "<SAS_In_Status>"
  Bus Selector4/8 -> Compare To Constant34/1  "<TCU_ActualGear>"
  Bus Selector4/9 -> Compare To Constant35/1  "<EPS_TrqLim_State>"
  Bus Selector4/10 -> Compare To Constant36/1  "<EPS_Trq_State>"
  Bus Selector4/11 -> Compare To Constant37/1  "<ESC_LatAcc_Valid>"
  Bus Selector4/12 -> Compare To Constant38/1  "<ESC_YawRate_Valid>"
  Bus Selector4/13 -> Compare To Constant39/1  "<ESC_LonAcc_Valid>"
  Compare To Constant30/1 -> Bus Creator1/5  "Event_FaulSASTrim"
  Compare To Constant31/1 -> Logical Operator5/2
  Compare To Constant28/1 -> Logical Operator5/1
  Bus Selector4/3 -> Compare To Constant31/1, Compare To Constant28/1  "<EPS_Error_State>"
  Compare To Constant32/1 -> Logical Operator6/1
  Compare To Constant33/1 -> Logical Operator6/2
  Compare To Constant35/1 -> Bus Creator1/8  "Event_FaulTrqLim"
  Compare To Constant34/1 -> Bus Creator1/7  "Event_FaulTCUGear"
  Compare To Constant36/1 -> Bus Creator1/9  "Event_FaulEPSTrqSt"
  Compare To Constant37/1 -> Bus Creator1/10  "Event_FaulLatAcc"
  Compare To Constant38/1 -> Bus Creator1/11  "Event_FaulYawRate"
  Compare To Constant39/1 -> Bus Creator1/12  "Event_FaulLonAcc"
  Bus Creator1/1 -> Bus Creator/2  "LKAS_ASWDTC_Status"
  Compare To Constant27/1 -> Bus Creator1/2  "Event_FaulEPSLKASt"
  Logical Operator5/1 -> Bus Creator1/3  "Event_FaulETATDA"
  Logical Operator6/1 -> Bus Creator1/6  "Event_FaulSWS"

== system LKAS/LKAS/LL/Human Machine Interface (HMI) ==
  HMI_stDACmode : Inport
  HMI_LDWWarn : Inport  Port=2
  HMI_LKA_STATE : Inport  Port=3
  HMI_LDW_STATE : Inport  Port=4
  HMI_R0_Quality : Inport  Port=5
  HMI_L0_Quality : Inport  Port=6
  HMI_EPSInfo : Inport  Port=7
  HMI_camera_common_fault : Inport  Port=8
  HMI_Front_Camera_Blocked : Inport  Port=9
  HMI_stFaultCSyn : Inport  Port=10
  Bus Creator2 : BusCreator  Inputs=7
  Cast To Single{,1..6} (7 alike) : DataTypeConversion  OutDataTypeStr=uint8
  HMI_Popup_Status : MATLAB Function  TreatAsAtomicUnit=on
  Hands_off_warning : MATLAB Function  TreatAsAtomicUnit=on
  LDW_Flag : MATLAB Function  TreatAsAtomicUnit=on
  LDW_Status_Display : MATLAB Function  TreatAsAtomicUnit=on
  LKA_Status_Display : MATLAB Function  TreatAsAtomicUnit=on
  LKA_action_indication : MATLAB Function  TreatAsAtomicUnit=on
  Subsystem : Subsystem
  Vehicle_Lane_Display : MATLAB Function  TreatAsAtomicUnit=on
  HMI_LDWLKA : Outport
  wires:
  HMI_LKA_STATE/1 -> Vehicle_Lane_Display/2(LKA_STATE), LKA_Status_Display/2(LKA_STATE), LDW_Flag/2(HMI_LKA_STATE), HMI_Popup_Status/2(LKA_STATE), LKA_action_indication/2(LKA_STATE)  "HMI_LKA_STATE"
  HMI_LDW_STATE/1 -> Subsystem/1(LDW_STATE), Vehicle_Lane_Display/3(LDW_STATE), LDW_Status_Display/2(LDW_STATE)  "HMI_LDW_STATE"
  Hands_off_warning/1(Hands_off_warning) -> Cast To Single4/1  "Hands_off_warning"
  LDW_Status_Display/1(LDW_Status_Display) -> Cast To Single1/1  "LDW_Status_Display"
  HMI_stFaultCSyn/1 -> HMI_Popup_Status/6(stFaultCSyn)  "HMI_stFaultCSyn"
  Bus Creator2/1 -> HMI_LDWLKA/1
  HMI_L0_Quality/1 -> Vehicle_Lane_Display/5(L0_Quality)  "HMI_L0_Quality"
  HMI_Popup_Status/1(HMI_Popup_Status) -> Cast To Single6/1  "HMI_Popup_Status"
  LKA_Status_Display/1(LKA_Status_Display) -> Cast To Single2/1  "LKA_Status_Display"
  HMI_stDACmode/1 -> Vehicle_Lane_Display/1(stDACmode), LDW_Status_Display/1(stDACmode), HMI_Popup_Status/1(stDACmode), LKA_action_indication/1(stDACmode), LDW_Flag/1(HMI_stDACmode), LKA_Status_Display/1(stDACmode)  "HMI_stDACmode"
  LDW_Flag/1(LDW_Flag) -> Cast To Single3/1  "LDW_Flag"
  HMI_Front_Camera_Blocked/1 -> HMI_Popup_Status/5(Front_Camera_Blocked)  "HMI_Front_Camera_Blocked"
  HMI_R0_Quality/1 -> Vehicle_Lane_Display/4(R0_Quality)  "HMI_R0_Quality"
  HMI_camera_common_fault/1 -> HMI_Popup_Status/4(camera_common_fault)  "HMI_camera_common_fault"
  LKA_action_indication/1(LKA_action_indication) -> Cast To Single5/1  "LKA_action_indication"
  Vehicle_Lane_Display/1(Vehicle_Lane_Display) -> Cast To Single/1  "Vehicle_Lane_Display"
  Cast To Single/1 -> Bus Creator2/1  "Vehicle_Lane_Display"
  Cast To Single1/1 -> Bus Creator2/2  "LDW_Status_Display"
  Cast To Single2/1 -> Bus Creator2/3  "LKA_Status_Display"
  Cast To Single3/1 -> Bus Creator2/4  "LDW_Flag"
  Cast To Single4/1 -> Bus Creator2/5  "Hands_off_warning"
  Cast To Single5/1 -> Bus Creator2/6  "LKA_action_indication"
  Cast To Single6/1 -> Bus Creator2/7  "HMI_Popup_Status"
  HMI_EPSInfo/1 -> Subsystem/2(EPSInfo)  "HMI_EPSInfo"
  Subsystem/1(HandsOff10s) -> HMI_Popup_Status/3(HandsOff)
  Subsystem/2(HandsOff15s) -> Hands_off_warning/1(HandsOff)
  HMI_LDWWarn/1 -> LDW_Flag/3(HMI_LDWWarnInfo)

== system LKAS/LKAS/LL/LL Inputs Mapping ==
  bsInInfo : Inport
  Bus Creator : BusCreator  Inputs=7
  Bus Selector : BusSelector  OutputSignals=bsMP5Info,bsLaneInfo,bsEPSInfo,bsVehMovInfo,bsSWAInfo,bsBCMInfo,bsPTState
  bsBCMInfo : Subsystem
  bsEPSInfo : Subsystem
  bsLaneInfo : Subsystem
  bsMP5Info : Subsystem
  bsPTState : Subsystem
  bsSWAInfo : Subsystem
  bsVehMovInfo : Subsystem
  bsInfo : Outport
  wires:
  bsSWAInfo/1(bsSWAInfoOut) -> Bus Creator/5  "bsSWAInfo"
  bsLaneInfo/1(bsLaneInfoOut) -> Bus Creator/2  "bsLaneInfo"
  bsPTState/1(bsPTStateOut) -> Bus Creator/7  "bsPTState"
  Bus Selector/7 -> bsPTState/1(bsPTStateIn)  "<bsPTState>"
  bsBCMInfo/1(bsBCMInfoOut) -> Bus Creator/6  "bsBCMInfo"
  bsMP5Info/1(bsMP5InfoOut) -> Bus Creator/1  "bsMP5Info"
  Bus Selector/1 -> bsMP5Info/1(bsMP5InfoIn)  "<bsMP5Info>"
  Bus Selector/6 -> bsBCMInfo/1(bsBCMInfoIn)  "<bsBCMInfo>"
  Bus Selector/5 -> bsSWAInfo/1(bsSWAInfoIn)  "<bsSWAInfo>"
  bsVehMovInfo/1(bsVehMovInfoOut) -> Bus Creator/4  "bsVehMovInfo"
  Bus Selector/4 -> bsVehMovInfo/1(bsVehMovInfoIn)  "<bsVehMovInfo>"
  bsEPSInfo/1(bsEPSInfoOut) -> Bus Creator/3  "bsEPSInfo"
  Bus Selector/3 -> bsEPSInfo/1(bsEPSInfoIn)  "<bsEPSInfo>"
  Bus Selector/2 -> bsLaneInfo/1(bsLaneInfoIn)  "<bsLaneInfo>"
  Bus Creator/1 -> bsInfo/1
  bsInInfo/1 -> Bus Selector/1

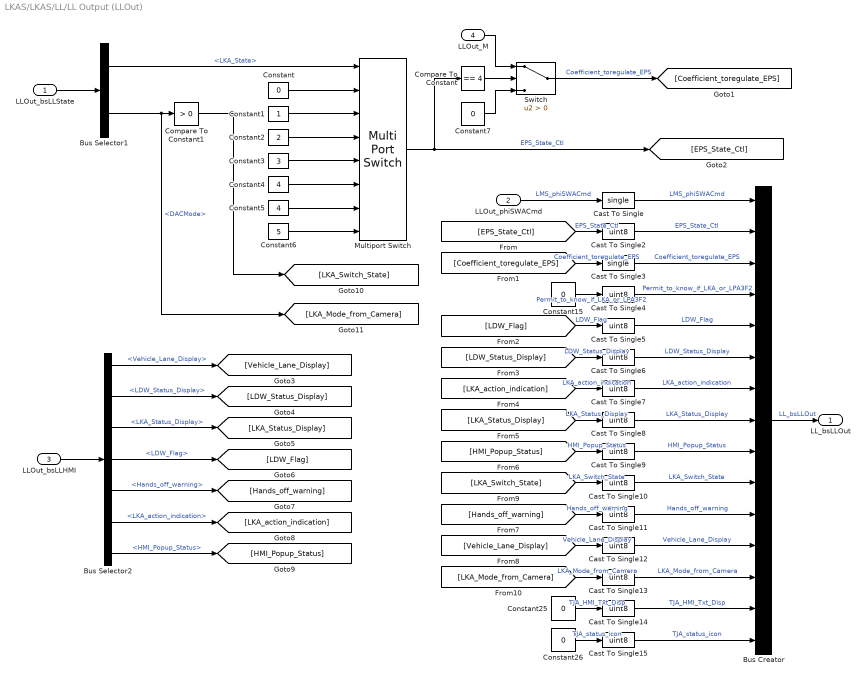
== system LKAS/LKAS/LL/LL Output (LLOut) ==
  LLOut_bsLLState : Inport
  LLOut_phiSWACmd : Inport  Port=2
  LLOut_bsLLHMI : Inport  Port=3
  LLOut_M : Inport  Port=4
  Bus Creator : BusCreator  Inputs=15
  Bus Selector1 : BusSelector  OutputSignals=LKA_State,DACMode
  Bus Selector2 : BusSelector  OutputSignals=Vehicle_Lane_Display,LDW_Status_Display,LKA_Status_Display,LDW_Flag,Hands_off_warning,LKA_action_indication,HMI_Popup_Status
  Cast To Single : DataTypeConversion  OutDataTypeStr=single
  Cast To Single{2,4..15} (13 alike) : DataTypeConversion  OutDataTypeStr=uint8
  Cast To Single3 : DataTypeConversion  OutDataTypeStr=single
  Compare To Constant : simulink/Logic and Bit Operations/Compare To Constant  relop===  const=4  OutDataTypeStr=boolean
  Compare To Constant1 : simulink/Logic and Bit Operations/Compare To Constant  relop=>  const=0  OutDataTypeStr=boolean
  Constant : Constant  Value=0  OutDataTypeStr=uint8
  Constant1 : Constant  OutDataTypeStr=uint8
  Constant15 : Constant  Value=0  OutDataTypeStr=uint16
  Constant2 : Constant  Value=2  OutDataTypeStr=uint8
  Constant25 : Constant  Value=0  OutDataTypeStr=uint8
  Constant26 : Constant  Value=0  OutDataTypeStr=uint8
  Constant3 : Constant  Value=3  OutDataTypeStr=uint8
  Constant4 : Constant  Value=4  OutDataTypeStr=uint8
  Constant5 : Constant  Value=4  OutDataTypeStr=uint8
  Constant6 : Constant  Value=5  OutDataTypeStr=uint8
  Constant7 : Constant  Value=0  OutDataTypeStr=single
  Multiport Switch : MultiPortSwitch  DataPortOrder=Zero-based contiguous  Inputs=7  zeroidx=on
  Switch : Switch  Criteria=u2 > Threshold
  LL_bsLLOut : Outport
  wires:
  Constant/1 -> Multiport Switch/2
  Constant5/1 -> Multiport Switch/7
  Cast To Single13/1 -> Bus Creator/13  "LKA_Mode_from_Camera"
  Cast To Single11/1 -> Bus Creator/11  "Hands_off_warning"
  Constant25/1 -> Cast To Single14/1  "TJA_HMI_Txt_Disp"
  LLOut_M/1 -> Switch/1
  Bus Selector2/2 -> [LDW_Status_Display]  "<LDW_Status_Display>"
  Cast To Single9/1 -> Bus Creator/9  "HMI_Popup_Status"
  Constant4/1 -> Multiport Switch/6
  Bus Selector2/6 -> [LKA_action_indication]  "<LKA_action_indication>"
  Cast To Single15/1 -> Bus Creator/15  "TJA_status_icon"
  Compare To Constant1/1 -> [LKA_Switch_State]
  LLOut_bsLLState/1 -> Bus Selector1/1
  Constant1/1 -> Multiport Switch/3
  Bus Selector2/1 -> [Vehicle_Lane_Display]  "<Vehicle_Lane_Display>"
  LLOut_bsLLHMI/1 -> Bus Selector2/1
  [EPS_State_Ctl] -> Cast To Single2/1  "EPS_State_Ctl"
  [LKA_Mode_from_Camera] -> Cast To Single13/1  "LKA_Mode_from_Camera"
  Cast To Single12/1 -> Bus Creator/12  "Vehicle_Lane_Display"
  Cast To Single6/1 -> Bus Creator/6  "LDW_Status_Display"
  Constant7/1 -> Switch/3
  Switch/1 -> [Coefficient_toregulate_EPS]  "Coefficient_toregulate_EPS"
  Multiport Switch/1 -> [EPS_State_Ctl], Compare To Constant/1  "EPS_State_Ctl"
  Bus Selector2/5 -> [Hands_off_warning]  "<Hands_off_warning>"
  Constant3/1 -> Multiport Switch/5
  Cast To Single3/1 -> Bus Creator/3  "Coefficient_toregulate_EPS"
  Cast To Single14/1 -> Bus Creator/14  "TJA_HMI_Txt_Disp"
  Bus Creator/1 -> LL_bsLLOut/1  "LL_bsLLOut"
  Cast To Single2/1 -> Bus Creator/2  "EPS_State_Ctl"
  Constant2/1 -> Multiport Switch/4
  Bus Selector1/2 -> [LKA_Mode_from_Camera], Compare To Constant1/1  "<DACMode>"
  Cast To Single10/1 -> Bus Creator/10  "LKA_Switch_State"
  Cast To Single4/1 -> Bus Creator/4  "Permit_to_know_if_LKA_or_LPA3F2"
  Cast To Single8/1 -> Bus Creator/8  "LKA_Status_Display"
  Constant26/1 -> Cast To Single15/1  "TJA_status_icon"
  [Hands_off_warning] -> Cast To Single11/1  "Hands_off_warning"
  [LKA_Switch_State] -> Cast To Single10/1  "LKA_Switch_State"
  [LDW_Status_Display] -> Cast To Single6/1  "LDW_Status_Display"
  Cast To Single/1 -> Bus Creator/1  "LMS_phiSWACmd"
  Bus Selector2/3 -> [LKA_Status_Display]  "<LKA_Status_Display>"
  LLOut_phiSWACmd/1 -> Cast To Single/1  "LMS_phiSWACmd"
  Bus Selector2/4 -> [LDW_Flag]  "<LDW_Flag>"
  [LKA_Status_Display] -> Cast To Single8/1  "LKA_Status_Display"
  Bus Selector1/1 -> Multiport Switch/1  "<LKA_State>"
  [HMI_Popup_Status] -> Cast To Single9/1  "HMI_Popup_Status"
  Cast To Single5/1 -> Bus Creator/5  "LDW_Flag"
  Constant6/1 -> Multiport Switch/8
  [LKA_action_indication] -> Cast To Single7/1  "LKA_action_indication"
  [Coefficient_toregulate_EPS] -> Cast To Single3/1  "Coefficient_toregulate_EPS"
  [LDW_Flag] -> Cast To Single5/1  "LDW_Flag"
  Constant15/1 -> Cast To Single4/1  "Permit_to_know_if_LKA_or_LPA3F2"
  [Vehicle_Lane_Display] -> Cast To Single12/1  "Vehicle_Lane_Display"
  Compare To Constant/1 -> Switch/2
  Bus Selector2/7 -> [HMI_Popup_Status]  "<HMI_Popup_Status>"
  Cast To Single7/1 -> Bus Creator/7  "LKA_action_indication"

== system LKAS/LKAS/LL/LLOn ==
  stDACMode : Inport
  bsInInfo : Inport  Port=2
  bsLLClb : Inport  Port=3
  bsSignalFault : Inport  Port=4
  states : EnablePort  StatesWhenEnabling=reset
      settings: AttributesFormatString=states = %<StatesWhenEnabling>
  Bus Selector : BusSelector  OutputSignals=bsLLSMConClb,bsLDWClb,bsLKAClb,bsConstantClb
  LDW : Subsystem  Description=|  TreatAsAtomicUnit=on
      | Block Name: Lane Departure Warning
      | Ab.: LDW
      | No.: 1.3.0.0
      | Rev: 0.0.1
      | Update Date: 19-3-26
  LKA : Subsystem  Description=|  TreatAsAtomicUnit=on
      | Block Name: Lane Keeping Assistance
      | Ab.: LKA
      | No.: 1.2.0.0
      | Rev: 0.0.1
      | Update Date: 19-5-13
  LKA Input Processing (LKAInP) : Subsystem
  LL State Determination (LLStateDet) : Subsystem
  LL_Mon : Subsystem
  bsLLState : Outport  OutputWhenDisabled=reset  InitialOutput=0
  LDW_Flag : Outport  Port=2
  phiSWACmd : Outport  Port=3  OutputWhenDisabled=reset  InitialOutput=0
  M : Outport  Port=4  OutputWhenDisabled=reset  InitialOutput=0
  LLMon : Outport  Port=5
  tag scope: LLClb_bsConstantClb=global, LLClb_bsLDWClb=global, LLClb_bsLKAClb=global, LLClb_bsLLSMConClb=global
  wires:
  [ActFlg] -> LKA Input Processing (LKAInP)/1(LKAInP_stLKAActvFlg)
  LL State Determination (LLStateDet)/2(LLStateDet_stLDWActvFlg) -> LDW/Enable, LDW/1(LDW_stLDWActvFlg)
  [LLClb_bsLLSMConClb] -> LL State Determination (LLStateDet)/4(LLStateDet_bsLLSMConClb)
  [LLClb_bsLKAClb] -> LKA Input Processing (LKAInP)/3(LKAInP_bsLKAClb)
  LL State Determination (LLStateDet)/1(LLStateDet_bsLLState) -> bsLLState/1
  [LLClb_bsLDWClb] -> LDW/3(LDW_bsLDWClb)
  LKA Input Processing (LKAInP)/1(LKAInP_bsLKAInPInfo) -> LKA/2(LKA_bsLKAInPInfo), LL State Determination (LLStateDet)/3(LLStateDet_bsLKAInPInfo)
  bsLLClb/1 -> Bus Selector/1
  [LLClb_bsLKAClb] -> LKA/3(LKA_bsLKAClb)
  Bus Selector/1 -> [LLClb_bsLLSMConClb]  "<bsLLSMConClb>"
  stDACMode/1 -> LL State Determination (LLStateDet)/1(LLStateDet_stDACMode)
  Bus Selector/3 -> [LLClb_bsLKAClb]  "<bsLKAClb>"
  Bus Selector/2 -> [LLClb_bsLDWClb]  "<bsLDWClb>"
  LL State Determination (LLStateDet)/3(LLStateDet_stLKAActvFlg) -> [ActFlg], LKA/Enable
  LDW/1(LDW_Flag) -> LDW_Flag/1  "LDW_Flag"
  bsInInfo/1 -> LKA Input Processing (LKAInP)/2(LKAInP_bsInInfoSyn), LL State Determination (LLStateDet)/2(LLStateDet_bsInInfoSyn), LKA/1(LKA_bsInInfoSyn), LDW/2(LDW_bsInInfoSyn)
  [ExitFlg] -> LL State Determination (LLStateDet)/5(LLStateDet_stExitFlg)
  Bus Selector/4 -> [LLClb_bsConstantClb]  "<bsConstantClb>"
  [LLClb_bsConstantClb] -> LKA/4(LKA_bsConstantClb)
  LKA/2(LKA_phiSWACmd) -> phiSWACmd/1  "OutputSWACmd"
  LKA/1(LKA_ExitFlg) -> [ExitFlg]
  bsSignalFault/1 -> LL State Determination (LLStateDet)/6(LLStateDet_SignalFault)
  LKA/3(LKA_M) -> M/1  "OutputM"
  LKA/4(LKAMon) -> [LKAMon]
  [LKAMon] -> LL_Mon/1(LKAMon)
  LL_Mon/1(LLMon) -> LLMon/1

== system LKAS/LKAS/LL/Subsystem ==
  bsInfo : Inport
  Bus Selector : BusSelector  OutputSignals=bsMP5Info.LKA_Main_Switch,bsMP5Info.LKA_Mode
  Divide : Product  Inputs=**  OutDataTypeStr=uint8
  On : Outport  OutDataTypeStr=uint8
  Mode : Outport  Port=2  OutDataTypeStr=uint8
  wires:
  Bus Selector/2 -> Divide/2  "<LKA_Mode>"
  bsInfo/1 -> Bus Selector/1
  Bus Selector/1 -> Divide/1, On/1  "<LKA_Main_Switch>"
  Divide/1 -> Mode/1

== system LKAS/LKAS/LLClb/ConstantClb ==
  Bus Creator : BusCreator  Inputs=6
  Data Type Conversion{2..4,6,13,22} (6 alike) : DataTypeConversion  OutDataTypeStr=single
  LKA_CarWidth=1.8 : Constant  Value=LKA_CarWidth
  LKA_SampleTime=0.01 : Constant  Value=LKA_SampleTime  OutDataTypeStr=single
  LKA_StrRatio_C=15.3 : Constant  Value=LKA_StrRatio_C
  LKA_Veh2CamL_C=1.56 : Constant  Value=LKA_Veh2CamL_C
  LKA_Veh2CamW_C=0.9 : Constant  Value=LKA_Veh2CamW_C  OutDataTypeStr=single
  LKA_WhlBaseL_C=2.65 : Constant  Value=LKA_WhlBaseL_C
  Switch{,1..3,11,19} (6 alike) : Switch  Criteria=u2 ~= 0  OutDataTypeStr=single
  ConstantClb : Outport
  wires:
  LKA_SampleTime=0.01/1 -> Switch19/3  "LKA_SampleTime"
  Data Type Conversion3/1 -> Switch19/1, Switch19/2
  Switch19/1 -> Bus Creator/1  "LKA_SampleTime"
  Switch2/1 -> Bus Creator/4  "LKA_WhlBaseL_C"
  Switch/1 -> Bus Creator/2  "LKA_Veh2CamW_C"
  Switch1/1 -> Bus Creator/3  "LKA_Veh2CamL_C"
  Switch11/1 -> Bus Creator/6  "LKA_CarWidth"
  Switch3/1 -> Bus Creator/5  "LKA_StrRatio_C"
  Bus Creator/1 -> ConstantClb/1
  LKA_CarWidth=1.8/1 -> Switch11/3  "LKA_CarWidth"
  Data Type Conversion22/1 -> Switch11/2, Switch11/1
  LKA_StrRatio_C=15.3/1 -> Switch3/3  "LKA_StrRatio_C"
  Data Type Conversion6/1 -> Switch3/2, Switch3/1
  Data Type Conversion4/1 -> Switch2/2, Switch2/1
  LKA_WhlBaseL_C=2.65/1 -> Switch2/3  "LKA_WhlBaseL_C"
  LKA_Veh2CamL_C=1.56/1 -> Switch1/3  "LKA_Veh2CamL_C"
  Data Type Conversion2/1 -> Switch1/2, Switch1/1
  Data Type Conversion13/1 -> Switch/2, Switch/1
  LKA_Veh2CamW_C=0.9/1 -> Switch/3  "LKA_Veh2CamW_C"

== system LKAS/LKAS/LLClb/LDWClb ==
  Bus Creator : BusCreator  Inputs=1
  Data Type Conversion6 : DataTypeConversion  OutDataTypeStr=single
  LL_LDWS_SUPPRESS_HEADING=2 : Constant  Value=LL_LDWS_SUPPRESS_HEADING  OutDataTypeStr=single
  Switch2 : Switch  Criteria=u2 ~= 0  OutDataTypeStr=single
  LDWClb : Outport
  wires:
  Data Type Conversion6/1 -> Switch2/2, Switch2/1
  LL_LDWS_SUPPRESS_HEADING=2/1 -> Switch2/3
  Switch2/1 -> Bus Creator/1  "LL_LDWS_SUPPRESS_HEADING"
  Bus Creator/1 -> LDWClb/1
